simulink model "oven"  (R2024b)
settings: Solver=VariableStepAuto  StartTime=0.0  StopTime=150  RelTol=1e-3
libraries: simulink x2, nesl_utility x1, simulink_extras x1
settings Model: Creator=29294  LastModifiedBy=29294
settings SolverCC: ZeroCrossAlgorithm=Adaptive

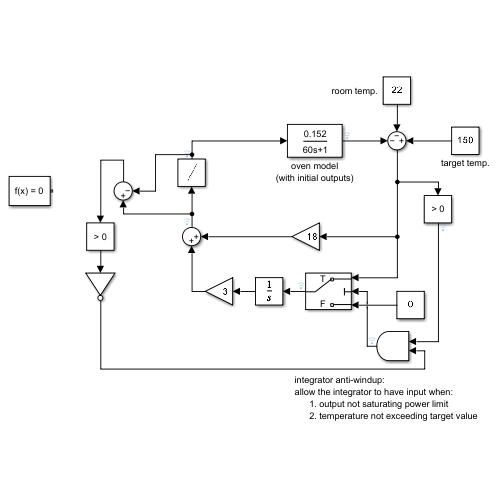
[thumbnail: Simulink's stored preview of the top-level diagram]
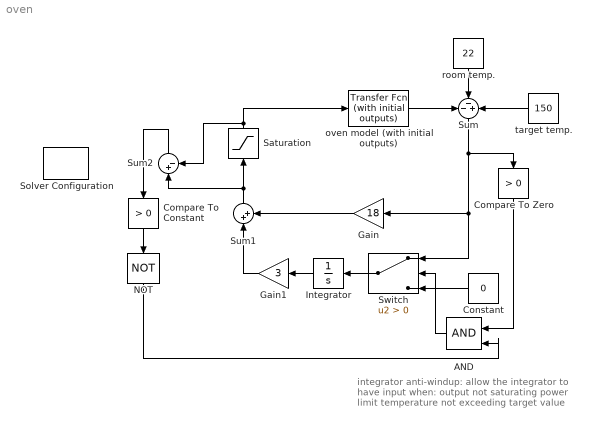
== system oven ==
  note: integrator anti-windup:
      | allow the integrator to have input when:
      | output not saturating power limit
      | temperature not exceeding target value
  AND : Logic  IconShape=distinctive  AllPortsSameDT=off
  Compare To Constant : simulink/Logic and Bit Operations/Compare To Constant  relop=>  const=0  OutDataTypeStr=boolean
  Compare To Zero : simulink/Logic and Bit Operations/Compare To Zero  relop=>  OutDataTypeStr=uint8
  Constant : Constant  Value=0
  Gain : Gain  Gain=18
  Gain1 : Gain  Gain=3
  Integrator : Integrator
  NOT : Logic  Operator=NOT  IconShape=distinctive  AllPortsSameDT=off
  Saturation : Saturate  UpperLimit=1500  LowerLimit=0
  Solver Configuration : nesl_utility/Solver Configuration  PhysicalDomain=network_engine_domain  SubClassName=solver  LeftPortType=input  RightPortType=generic  Tones=[]  Harmonics=[]  SimulateNoise=off  Profile=off  UseLocalSampling=off  EnableSwitchedLinearOptims=on  FrequencyDomain=off  UseCCode=off  RelTol=0.001  AbsTol=0.001  MinStep=1e-09  ToWorkspace=off  RevertToSquareIcSolve=off  NumHomotopyIterations=100  PhasorMode=off  PhasorModeNumHarmonics=1  ConsistencySolver=NEWTON_XTOL_AFTER_FTOL  IndexReductionMethod=DerivativeReplacement  DoDC=off  ResidualTolerance=1e-09  ConsistencyTolSource=GLOBAL  ConsistencyAbsTol=0.001  ConsistencyRelTol=0.001  ConsistencyTolFactor=0.001  UseLocalSolver=off  LocalSolverChoice=NE_BACKWARD_EULER_ADVANCER  ResolveIndetEquations=on  FunctionEvalNumThread=1  LocalSolverSampleTime=0.001  DoFixedCost=off  MaxNonlinIter=3  MaxModeIter=2  ComputeImpulses=off  ImpulseIterations=2  LinearAlgebra=auto  LinearAlgebraNumThread=0  EquationFormulation=NE_TIME_EF  DelaysMemoryBudget=1024  AutomaticFiltering=on  FilteringTimeConstant=0.001  PartitionStorageMethod=AS_NEEDED  PartitionMemoryBudget=1024  PartitionMethod=ROBUST  MultibodyUseLocalSolver=off  MultibodyLocalSolverChoice=ODE1  MultibodyLocalSolverSampleTime=0.001
  Sum : Sum  Inputs=--+
  Sum1 : Sum  Inputs=|++
  Sum2 : Sum  Inputs=|+-
  Switch : Switch  Criteria=u2 > Threshold  SaturateOnIntegerOverflow=off  InputSameDT=off
  oven model (with initial outputs) : simulink_extras/Additional Linear/Transfer Fcn (with initial outputs)  N=[0.152]  D="[60  1]"  Y0=22  U0=0
  room temp. : Constant  Value=22
  target temp. : Constant  Value=150
  wires:
  oven model (with initial outputs)/1 -> Sum/1
  target temp./1 -> Sum/3
  Sum/1 -> Compare To Zero/1, Switch/1, Gain/1
  Integrator/1 -> Gain1/1
  Gain/1 -> Sum1/2
  Sum1/1 -> Sum2/1, Saturation/1
  Saturation/1 -> Sum2/2, oven model (with initial outputs)/1
  room temp./1 -> Sum/2
  Gain1/1 -> Sum1/1
  Constant/1 -> Switch/3
  Compare To Zero/1 -> AND/1
  AND/1 -> Switch/2
  Sum2/1 -> Compare To Constant/1
  Compare To Constant/1 -> NOT/1
  NOT/1 -> AND/2
  Switch/1 -> Integrator/1
